simulink model "ADCCalibration_MDL"  (R2016b)
settings: Solver=FixedStepAuto  StartTime=0.0  StopTime=20  FixedStep=0.02  RelTol=1e-3
libraries: MSCubeLibrary x2
settings Model: SimulationMode=external  Creator=ich  LastModifiedBy=ich
settings OptimizationCC: MaxStackSize=64
settings DebuggingCC: ParameterTunabilityLossMsg=error
settings HardwareCC: ProdBitPerPointer=32  ProdBitPerSizeT=32  ProdBitPerPtrDiffT=32  ProdLargestAtomicInteger=Long  ProdLargestAtomicFloat=Double  ProdWordSize=32  ProdHWDeviceType=ARM Compatible->ARM Cortex
settings RTWCC: SystemTargetFile=ert.tlc  HardwareBoard=MSCubeBBB  TLCOptions="-aInlineSetEventsForThisBaseRateFcn=TLC_FALSE -aSuppressMultiTaskScheduler=TLC_FALSE  -aRateBasedStepFcn=0"  TemplateMakefile=ert_default_tmf  Description=Embedded Coder  GenerateReport=on  Toolchain=Linaro Toolchain v4.8  IncludeHyperlinkInReport=on  LaunchReport=on  GenerateTraceInfo=on  GenerateTraceReport=on  GenerateTraceReportSl=on  GenerateTraceReportSf=on  GenerateTraceReportEml=on
settings CodeAppCC: ForceParamTrailComments=on  IgnoreCustomStorageClasses=off  OperatorAnnotations=on  SimulinkDataObjDesc=on  SFDataObjDesc=on  MATLABFcnDesc=on  InsertBlockDesc=on  MATLABSourceComments=on

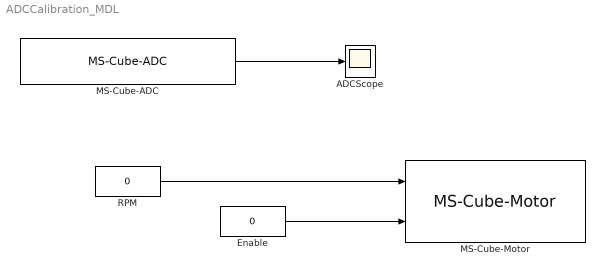
== system ADCCalibration_MDL ==
  ADCScope : Scope
  Enable : Constant  Value=0  OutDataTypeStr=boolean
  MS-Cube-ADC : MSCubeLibrary/MS-Cube-ADC
  MS-Cube-Motor : MSCubeLibrary/MS-Cube-Motor
  RPM : Constant  Value=0  OutDataTypeStr=single
  wires:
  MS-Cube-ADC/1 -> ADCScope/1
  RPM/1 -> MS-Cube-Motor/1
  Enable/1 -> MS-Cube-Motor/2
